simulink model "lab3mm1_2"  (R2018b)
settings: Solver=VariableStepAuto  StartTime=0.0  StopTime=1000000  RelTol=1e-3  EnableMultiTasking=on
undefined symbols (not defined in the file): m, n
libraries: simulink x2
settings Model: Creator=The MathWorks, Inc.  LastModifiedBy=vano7
settings DataIOCC: LimitDataPoints=on  SaveFormat=Array
settings OptimizationCC: LifeSpan=inf
settings DebuggingCC: AllowSymbolicDim=off  SFUnexpectedBacktrackingDiag=warning  SFNoUnconditionalDefaultTransitionDiag=warning  SFExecutionAtInitializationDiag=none
settings ModelReferenceCC: PropagateSignalLabelsOutOfModel=off
settings SFSimCC: SimUseLocalCustomCode=off
settings RTWCC: RTWUseLocalCustomCode=off
settings CodeAppCC: StateflowObjectComments=on
settings GRTTargetCC: TargetLangStandard=C89/C90 (ANSI)  GeneratePreprocessorConditionals=Disable all
settings ConfigComp: CovMetricSettings=dw  CovHtmlReporting=on  CovSaveCumulativeToWorkspaceVar=on  CovSaveSingleToWorkspaceVar=on  CovExternalEMLEnable=off  CovSFcnEnable=off

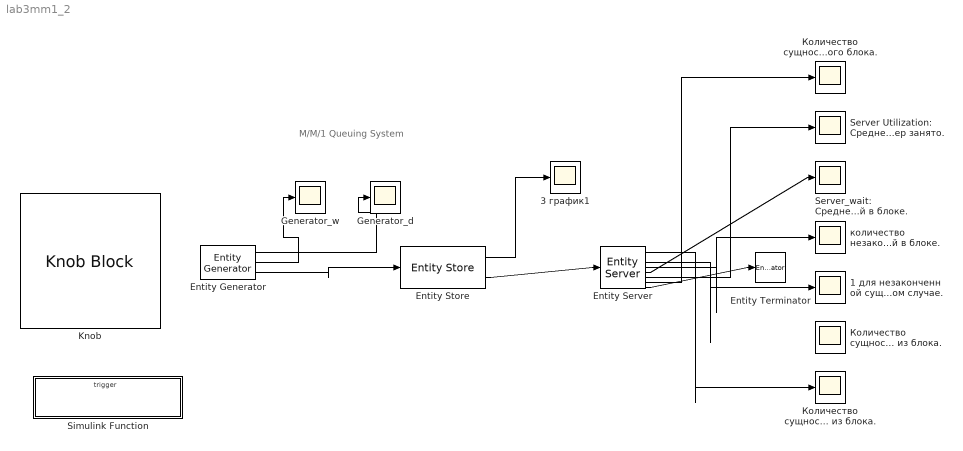
== system lab3mm1_2 ==
  note: M/M/1 Queuing System
  " 1 для незаконченной сущности в блоке и 0 в противном случае." : Scope
  3 график1 : Scope
  Entity Generator : EntityGenerator  OutputPortMessageModes=n,n,m  TimeSource=MATLAB action  IntergenerationTimeAction=dt = exponentialArrivalTime();  NumberEntitiesDeparted=on  AverageIntergenerationTime=on  EntityType=Structured  EntityTypeName=Entity
      settings: OutputPortMap=o0,o2,o3
  Entity Server : EntityServer  InputPortMessageModes=m  OutputPortMessageModes=n,n,n,n,n,n,n,m  Capacity=1  ServiceTimeValue=1  ServiceTimeAction=|  NumberEntitiesDeparted=on  NumberEntitiesInBlock=on  PendingEntityPresentInBlock=on  NumberEntitiesPending=on  AverageWait=on  Utilization=on  NumEntitiesExtracted=on
      | % Exponential service time with rate 1
      | mean = 1;
      | dt   = -mean * log(1 - rand());
      settings: OutputPortMap=o0,o1,o2,o3,o4,o5,o12,o9
  Entity Store : EntityStore  InputPortMessageModes=m  OutputPortMessageModes=n,m  Capacity=100000000  AverageWait=on
      settings: OutputPortMap=o2,o4
  Entity Terminator : EntityTerminator  InputPortMessageModes=m
  Generator_d : Scope
  Generator_w : Scope
  Knob : KnobBlock  WebBlockId=170  ScaleMin=0.01  ScaleMax=0.999
  Server Utilization: Среднее время сервер занято. : Scope
  "Server_wait: Среднее время ожидания для сущностей в блоке. " : Scope
  Simulink Function : Subsystem  TreatAsAtomicUnit=on
  "Количество сущностей, которые вытащены этого блока. " : Scope
  "Количество сущностей, которые еще не отбыли из блока. " : Scope
  "Количество сущностей, которые отбыли из блока." : Scope
  количество незаконченных сущностей в блоке. : Scope
  wires:
  Entity Generator/3 -> Entity Store/1
  Entity Store/2 -> Entity Server/1
  Entity Server/8 -> Entity Terminator/1
  Entity Server/6 -> Server Utilization: Среднее время сервер занято./1
  Entity Generator/2 -> Generator_w/1
  Entity Server/5 -> "Server_wait: Среднее время ожидания для сущностей в блоке. "/1
  Entity Server/7 -> "Количество сущностей, которые вытащены этого блока. "/1
  Entity Server/4 -> количество незаконченных сущностей в блоке./1
  Entity Server/3 -> " 1 для незаконченной сущности в блоке и 0 в противном случае."/1
  Entity Server/1 -> "Количество сущностей, которые отбыли из блока."/1
  Entity Generator/1 -> Generator_d/1
  Entity Store/1 -> 3 график1/1

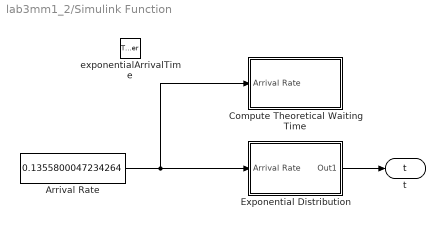
== system lab3mm1_2/Simulink Function ==
  exponentialArrivalTime : TriggerPort  TriggerType=function-call  IsSimulinkFunction=on  FunctionName=exponentialArrivalTime  VariantControl=Variant
  Arrival Rate : Constant  Value=0.1355800047234264  SampleTime=-1
  Compute Theoretical Waiting Time : Subsystem
  Exponential Distribution : Subsystem
  t : ArgOut  DisableCoverage=on  ArgumentName=t
  wires:
  Arrival Rate/1 -> Compute Theoretical Waiting Time/1(Arrival Rate), Exponential Distribution/1(Arrival Rate)
  Exponential Distribution/1(Out1) -> t/1

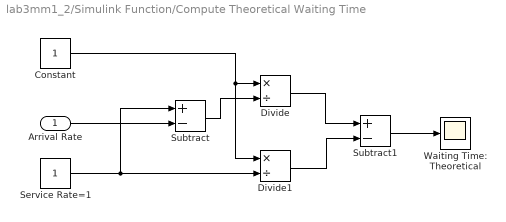
== system lab3mm1_2/Simulink Function/Compute Theoretical Waiting Time ==
  Arrival Rate : Inport
  Constant : Constant
  Divide : Product  Inputs=*/
  Divide1 : Product  Inputs=*/
  Service Rate=1 : Constant
  Subtract : Sum  Inputs=+-
  Subtract1 : Sum  Inputs=+-
  Waiting Time: Theoretical : Scope
  wires:
  Arrival Rate/1 -> Subtract/2
  Subtract1/1 -> Waiting Time: Theoretical/1
  Divide1/1 -> Subtract1/2
  Divide/1 -> Subtract1/1
  Subtract/1 -> Divide/2
  Constant/1 -> Divide1/1, Divide/1
  Service Rate=1/1 -> Subtract/1, Divide1/2

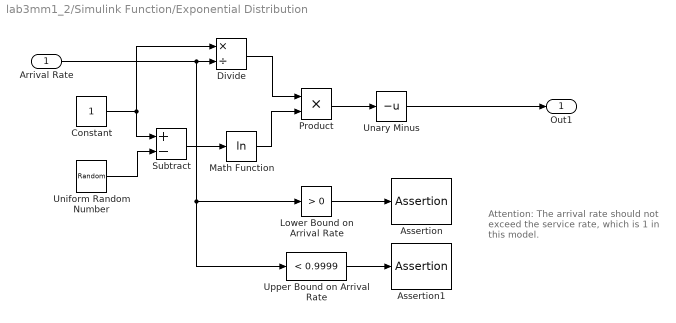
== system lab3mm1_2/Simulink Function/Exponential Distribution ==
  note: Attention: The arrival rate
      | should not exceed the service
      | rate, which is 1 in this model.
  Arrival Rate : Inport
  Assertion : Assertion
  Assertion1 : Assertion
  Constant : Constant
  Divide : Product  Inputs=*/
  Lower Bound on Arrival Rate : simulink/Logic and Bit Operations/Compare To Constant  relop=>  const=0  OutDataTypeStr=uint8  ZeroCross=off
  Math Function : Math  Operator=log  SaturateOnIntegerOverflow=on
  Product : Product  RndMeth=Zero
  Subtract : Sum  Inputs=+-
  Unary Minus : UnaryMinus
  Uniform Random Number : UniformRandomNumber  Minimum=0  Seed=12345
  "Upper Bound on Arrival Rate " : simulink/Logic and Bit Operations/Compare To Constant  relop=<  const=0.9999  OutDataTypeStr=uint8  ZeroCross=off
  Out1 : Outport
  wires:
  Arrival Rate/1 -> Divide/2, Lower Bound on Arrival Rate/1, "Upper Bound on Arrival Rate "/1
  Unary Minus/1 -> Out1/1
  Product/1 -> Unary Minus/1
  Math Function/1 -> Product/2
  Divide/1 -> Product/1
  Constant/1 -> Divide/1, Subtract/1
  Uniform Random Number/1 -> Subtract/2
  Lower Bound on Arrival Rate/1 -> Assertion/1
  "Upper Bound on Arrival Rate "/1 -> Assertion1/1
  Subtract/1 -> Math Function/1
